simulink model "simulering_ROV_STA_controller"  (R2020a)
settings: Solver=ode45  StartTime=0.0  StopTime=t_sim  RelTol=1e-3
values from neighbouring files (symbols this model uses):
  alpha_los = atan2(y_los-y_start,x_los-x_start)    [run_simulation_SM_controller.m]    (also in run_simulation_STA_controller.m; run_simulation_dp_model.m)
  alpha_m_psi = 1    [run_simulation_STA_controller.m]    (also in tuning_STA_controller.m = 1.5)
  alpha_m_u = 1    [run_simulation_STA_controller.m]    (also in tuning_STA_controller.m = 1.5)
  alpha_m_v = 1    [run_simulation_STA_controller.m]    (also in tuning_STA_controller.m = 1.5)
  alpha_m_w = 1    [run_simulation_STA_controller.m]    (also in tuning_STA_controller.m = 1.5)
  B_aug = [b11 b12 b13 b14 b15 b16 ... (first row only)    [constants.m]
  B_psinv_aug = B_aug'/(B_aug*B_aug')    [constants.m]
  d_11 = 250    [constants.m]    (also in constants_dp_model.m; constants_model_coriolis.m; constants_process_model.m)
  d_22 = 200    [constants.m]    (also in constants_dp_model.m; constants_model_coriolis.m; constants_process_model.m)
  d_33 = 175    [constants.m]    (also in constants_dp_model.m; constants_model_coriolis.m; constants_process_model.m)
  d_66 = 15    [constants.m]    (also in constants_process_model.m)
  d_n11 = 350    [constants.m]
  d_n22 = 350    [constants.m]
  d_n33 = 400    [constants.m]
  d_n66 = 75    [constants.m]
  Delta = 25    [plot_simulation_feedback.m]    (also in run_simulation.m; run_simulation_SM_controller.m; run_simulation_STA_controller.m; run_simulation_dp_model.m)
  epsilon_psi = 1    [run_simulation_STA_controller.m]    (also in tuning_STA_controller.m = 0.0001)
  epsilon_u = 1    [run_simulation_STA_controller.m]    (also in tuning_STA_controller.m = 0.0001)
  epsilon_v = 1    [run_simulation_STA_controller.m]    (also in tuning_STA_controller.m = 0.0001)
  epsilon_w = 1    [run_simulation_STA_controller.m]    (also in tuning_STA_controller.m = 0.0001)
  g_z = 9.81    [run_simulation_FL_controller.m]    (also in run_simulation_PID_controller.m = 0.91; run_simulation_SM_controller.m = 0.91; run_simulation_STA_controller.m = 0.91; run_simulation_dp_model.m = 0.91)
  gam_psi = 1    [run_simulation_STA_controller.m]    (also in tuning_STA_controller.m)
  gam_u = 1    [run_simulation_STA_controller.m]    (also in tuning_STA_controller.m)
  gam_v = 1    [run_simulation_STA_controller.m]    (also in tuning_STA_controller.m)
  gam_w = 1    [run_simulation_STA_controller.m]    (also in tuning_STA_controller.m)
  gamma_r = 0.1    [run_simulation_FL_controller.m]    (also in run_simulation_PID_controller.m; run_simulation_SM_controller.m; run_simulation_STA_controller.m; run_simulation_feedback_linearizing.m)
  gamma_u = 0.1    [run_simulation_FL_controller.m]    (also in run_simulation_PID_controller.m; run_simulation_SM_controller.m; run_simulation_STA_controller.m; run_simulation_feedback_linearizing.m)
  gamma_v = 0.1    [run_simulation_FL_controller.m]    (also in run_simulation_PID_controller.m; run_simulation_SM_controller.m; run_simulation_STA_controller.m; run_simulation_feedback_linearizing.m)
  lambda = d_44    [run_simulation_FL_controller.m]    (also in run_simulation_PID_controller.m = 1; run_simulation_SM_controller.m = 1; run_simulation_STA_controller.m = 1; run_simulation_feedback_linearizing.m = 1)
  lambda_psi = 1    [run_simulation_SM_controller.m]    (also in run_simulation_STA_controller.m; tuning_SM_controller.m; tuning_STA_controller.m = 0.5)
  lambda_u = 0.5    [run_simulation_SM_controller.m]    (also in run_simulation_STA_controller.m = 1; tuning_SM_controller.m; tuning_STA_controller.m = 10)
  lambda_v = 0.5    [run_simulation_SM_controller.m]    (also in run_simulation_STA_controller.m = 1; tuning_SM_controller.m; tuning_STA_controller.m = 10)
  lambda_w = 1    [run_simulation_STA_controller.m]    (also in tuning_STA_controller.m = 0.5)
  m_11 = m_RB11+m_A11    (= 144)    [constants.m]    (also in constants_dp_model.m; constants_model_coriolis.m; constants_process_model.m)
  m_22 = m_RB22+m_A22    (= 162)    [constants.m]    (also in constants_dp_model.m; constants_model_coriolis.m; constants_process_model.m)
  m_66 = m_RB66+m_A66    (= 18.2)    [constants.m]    (also in constants_process_model.m)
  m_A11 = 54    [constants.m]    (also in constants_dp_model.m; constants_model_coriolis.m; constants_process_model.m)
  m_A22 = 72    [constants.m]    (also in constants_dp_model.m; constants_model_coriolis.m; constants_process_model.m)
  m_A33 = 360    [constants.m]    (also in constants_dp_model.m; constants_model_coriolis.m; constants_process_model.m)
  m_A66 = 5.2    [constants.m]    (also in constants_process_model.m)
  m_RB11 = 90    [constants.m]    (also in constants_dp_model.m; constants_model_coriolis.m; constants_process_model.m)
  m_RB22 = 90    [constants.m]    (also in constants_dp_model.m; constants_model_coriolis.m; constants_process_model.m)
  m_RB33 = 90    [constants.m]    (also in constants_dp_model.m; constants_model_coriolis.m; constants_process_model.m)
  m_RB66 = 13    [constants.m]    (also in constants_process_model.m)
  omega_psi = 1    [run_simulation_STA_controller.m]    (also in tuning_STA_controller.m = 0.001)
  omega_ref = 1.5    [run_simulation.m]    (also in run_simulation_FL_controller.m = 0.4; run_simulation_PID_controller.m = 0.4; run_simulation_SM_controller.m; run_simulation_STA_controller.m = 0.4)
  omega_u = 1    [run_simulation_STA_controller.m]    (also in tuning_STA_controller.m = 0.01)
  omega_v = 1    [run_simulation_STA_controller.m]    (also in tuning_STA_controller.m = 0.01)
  omega_w = 1    [run_simulation_STA_controller.m]    (also in tuning_STA_controller.m = 0.01)
  psi0 = deg2rad(psi0)    [constants.m]    (also in constants_dp_model.m; constants_model_coriolis.m; constants_process_model.m)
  r0 = 0    [constants.m]    (also in constants_dp_model.m; constants_model_coriolis.m; constants_process_model.m)
  T_ref = 0.2    [run_simulation.m]    (also in run_simulation_FL_controller.m; run_simulation_PID_controller.m; run_simulation_SM_controller.m; run_simulation_STA_controller.m)
  tau_r_max = sqrt(torque_co'*torque_co)    [constants.m]    (also in constants_dp_model.m; constants_model_coriolis.m; constants_process_model.m; run_simulation_feedback_linearizing.m = sqrt(torque_co'*torque_co)/(m_A33+m_RB33))
  tau_u_max = (F_max*cos(alpha1)+F_max*cos(alpha2)+F_max*cos(alpha3)+F_max*cos(alpha4))    [constants.m]    (also in constants_dp_model.m; constants_model_coriolis.m; constants_process_model.m; run_simulation_feedback_linearizing.m = (F_max*cos(alpha1)+F_max*cos(alpha2)+F_max*cos(alpha3)+F_max)
  tau_v_max = (F_max*sin(alpha1)-F_max*sin(alpha2)+F_max*sin(alpha3)-F_max*sin(alpha4))    [constants.m]    (also in constants_dp_model.m; constants_model_coriolis.m; constants_process_model.m; run_simulation_feedback_linearizing.m = (F_max*sin(alpha1)-F_max*sin(alpha2)+F_max*sin(alpha3)-F_max)
  tau_w_max = 2*F_max    (= 240)    [constants.m]    (also in constants_dp_model.m; constants_model_coriolis.m; constants_process_model.m)
  u0 = 0    [constants.m]    (also in constants_dp_model.m; constants_model_coriolis.m; constants_process_model.m)
  u_r = 0.14    [run_simulation.m]    (also in run_simulation_FL_controller.m = 0.2; run_simulation_PID_controller.m = 0.2; run_simulation_SM_controller.m; run_simulation_STA_controller.m = 0.2)
  v0 = 0    [constants.m]    (also in constants_dp_model.m; constants_model_coriolis.m; constants_process_model.m)
  v_r = 0.14    [run_simulation.m]    (also in run_simulation_FL_controller.m = 0; run_simulation_PID_controller.m = 0; run_simulation_SM_controller.m; run_simulation_STA_controller.m = 0)
  V_x_mat = load('Vx_disturbance.mat').u    [run_simulation_SM_controller.m]    (also in run_simulation_STA_controller.m; run_simulation_dp_model.m)
  V_y_mat = load('Vy_disturbance.mat').v    [run_simulation_SM_controller.m]    (also in run_simulation_STA_controller.m; run_simulation_dp_model.m)
  w0 = 0    [constants.m]    (also in constants_dp_model.m; constants_model_coriolis.m; constants_process_model.m)
  x0 = -2*50    (= -100)    [constants.m]    (also in constants_dp_model.m = 0; constants_model_coriolis.m = 0; constants_process_model.m = 0)
  x_start = -2*50    (= -100)    [plot_simulation_feedback.m]    (also in run_simulation_SM_controller.m; run_simulation_STA_controller.m; run_simulation_dp_model.m)
  y0 = 0    [constants.m]    (also in constants_dp_model.m; constants_model_coriolis.m; constants_process_model.m)
  y_start = 1*80    (= 80)    [plot_simulation_feedback.m]    (also in run_simulation_SM_controller.m; run_simulation_STA_controller.m = 50; run_simulation_dp_model.m)
  z0 = 0    [constants.m]    (also in constants_dp_model.m; constants_model_coriolis.m; constants_process_model.m)
  z_r = 10    [run_simulation.m]    (also in run_simulation_FL_controller.m = 1; run_simulation_PID_controller.m = 1; run_simulation_SM_controller.m; run_simulation_STA_controller.m = 1)
  zeta_ref = 1    [run_simulation.m]    (also in run_simulation_FL_controller.m; run_simulation_PID_controller.m; run_simulation_SM_controller.m; run_simulation_STA_controller.m)
settings Model: Creator=kenng  LastModifiedBy=kenng

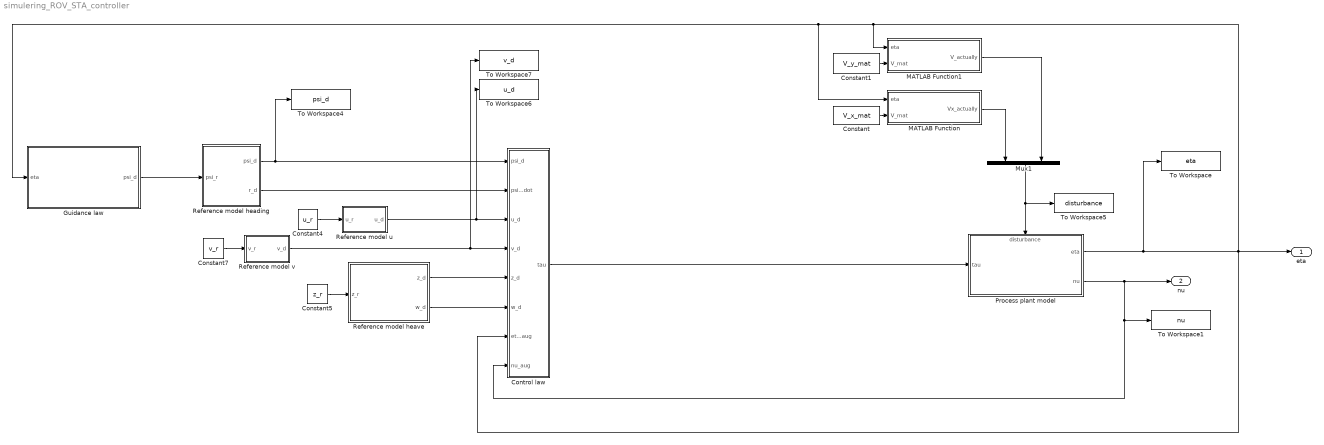
== system simulering_ROV_STA_controller ==
  Constant : Constant  Value=V_x_mat
  Constant1 : Constant  Value=V_y_mat
  Constant4 : Constant  Value=u_r
  Constant5 : Constant  Value=z_r
  Constant7 : Constant  Value=v_r
  Control law : Subsystem
  Guidance law : Subsystem
  MATLAB Function : MATLAB Function  TreatAsAtomicUnit=on
  MATLAB Function1 : MATLAB Function  TreatAsAtomicUnit=on
  Mux1 : Mux  Inputs=2
  Process plant model : Subsystem
      settings: PortSchema="{\"entries\":[{\"content\":{\"sides\":[{\"content\":{\"connectorIds\":[\"In1\"]},\"type\":\"ConnectorPlacement.EquallySpacedRectSide\",\"uuid\":\"e717a587-3200-458e-ba24-dd41565550b9\"},{\"content\":{\"connectorIds\":[\"Out1\",\"Out2\"],\"side\":\"RIGHT\"},\"type\":\"ConnectorPlacement.EquallySpacedRectSide\",\"uuid\":\"302c9cc9-c34e-45c2-bf93-40982187bd66\"},{\"content\":{\"connectorIds\":[\"In2\"],\"side\":\"TOP\"},\"type\":\"ConnectorPlacement.EquallySpacedRectSide\",\"uuid\":\"4b1c13ad-6fa1-447d-8a08-ad292496a8ea\"}]},\"type\":\"ConnectorPlacement.EquallySpacedConnector\",\"uuid\":\"78ff5622-69b9-4402-ac71-5e2cc2861626\"}],\"packageUris\":[\"http://schema.mathworks.com/mf0/Connector/19700101\"],\"version\":\"1.0\"}"
  Reference model heading : Subsystem
  Reference model heave : Subsystem
  Reference model u : Subsystem
  Reference model v : Subsystem
  To Workspace : ToWorkspace  VariableName=eta  SaveFormat=Structure With Time  SampleTime=-1
  To Workspace1 : ToWorkspace  VariableName=nu  SaveFormat=Structure With Time  SampleTime=-1
  To Workspace4 : ToWorkspace  VariableName=psi_d  SaveFormat=Structure With Time  SampleTime=-1
  To Workspace5 : ToWorkspace  VariableName=disturbance  SaveFormat=Structure With Time  SampleTime=-1
  To Workspace6 : ToWorkspace  VariableName=u_d  SaveFormat=Structure With Time  SampleTime=-1
  To Workspace7 : ToWorkspace  VariableName=v_d  SaveFormat=Structure With Time  SampleTime=-1
  eta : Outport
  nu : Outport  Port=2
  wires:
  Process plant model/2(nu) -> nu/1, To Workspace1/1, Control law/8(nu_aug)
  Mux1/1 -> Process plant model/2(disturbance), To Workspace5/1
  MATLAB Function/1(Vx_actually) -> Mux1/1
  MATLAB Function1/1(V_actually) -> Mux1/2
  Reference model heave/1(z_d) -> Control law/5(z_d)
  Reference model u/1(u_d) -> To Workspace6/1, Control law/3(u_d)
  Constant7/1 -> Reference model v/1(v_r)
  Guidance law/1(psi_d) -> Reference model heading/1(psi_r)
  Reference model heave/2(w_d) -> Control law/6(w_d)
  Reference model heading/1(psi_d) -> Control law/1(psi_d), To Workspace4/1
  Constant4/1 -> Reference model u/1(u_r)
  Reference model v/1(v_d) -> To Workspace7/1, Control law/4(v_d)
  Reference model heading/2(r_d) -> Control law/2(psi_d_dot)
  Constant5/1 -> Reference model heave/1(z_r)
  Control law/1(tau) -> Process plant model/1(tau)
  Constant1/1 -> MATLAB Function1/2(V_mat)
  Process plant model/1(eta) -> To Workspace/1, MATLAB Function1/1(eta), Guidance law/1(eta), MATLAB Function/1(eta), Control law/7(eta_aug), eta/1
  Constant/1 -> MATLAB Function/2(V_mat)

== system simulering_ROV_STA_controller/Control law ==
  psi_d : Inport
  psi_d_dot : Inport  Port=2
  u_d : Inport  Port=3
  v_d : Inport  Port=4
  z_d : Inport  Port=5
  w_d : Inport  Port=6
  eta_aug : Inport  Port=7
  nu_aug : Inport  Port=8
  Adaptive law r : Subsystem
  Adaptive law u : Subsystem
  Adaptive law v : Subsystem
  Heave controller : Subsystem
  Mux : Mux
  Surge controller : Subsystem
  Sway controller : Subsystem
  To Workspace : ToWorkspace  VariableName=V_yv_hat  SaveFormat=Structure With Time  SampleTime=-1
  To Workspace1 : ToWorkspace  VariableName=V_yu_hat  SaveFormat=Structure With Time  SampleTime=-1
  To Workspace2 : ToWorkspace  VariableName=V_xv_hat  SaveFormat=Structure With Time  SampleTime=-1
  To Workspace3 : ToWorkspace  VariableName=V_xu_hat  SaveFormat=Structure With Time  SampleTime=-1
  To Workspace4 : ToWorkspace  VariableName=V_xr_hat  SaveFormat=Structure With Time  SampleTime=-1
  To Workspace5 : ToWorkspace  VariableName=V_yr_hat  SaveFormat=Structure With Time  SampleTime=-1
  To Workspace6 : ToWorkspace  VariableName=V_xr_hat_sq  SaveFormat=Structure With Time  SampleTime=-1
  To Workspace7 : ToWorkspace  VariableName=V_yr_hat_sq  SaveFormat=Structure With Time  SampleTime=-1
  To Workspace8 : ToWorkspace  VariableName=V_xyr_hat  SaveFormat=Structure With Time  SampleTime=-1
  Yaw controller : Subsystem
  tau : Outport
  wires:
  Heave controller/1(tau_w) -> Mux/3
  Mux/1 -> tau/1
  u_d/1 -> Surge controller/1(u_d), Adaptive law u/3(u_d)
  v_d/1 -> Adaptive law v/3(v_d), Sway controller/1(v_d)
  z_d/1 -> Heave controller/1(z_d)
  Adaptive law u/2(V_y_u_hat) -> To Workspace1/1
  Adaptive law u/1(V_x_u_hat) -> To Workspace3/1
  Adaptive law v/1(V_yv_hat) -> To Workspace/1
  Adaptive law v/2(V_xv_hat) -> To Workspace2/1
  Adaptive law r/1(V_xr_hat) -> To Workspace4/1
  Adaptive law r/2(V_yr_hat) -> To Workspace5/1
  Adaptive law r/3(V_xr_hat_sq) -> To Workspace6/1
  Adaptive law r/4(V_yr_hat_sq) -> To Workspace7/1
  Adaptive law r/5(V_xyr_hat) -> To Workspace8/1
  [psi_d] -> Adaptive law r/3(psi_d)
  psi_d_dot/1 -> Yaw controller/4(psi_d_dot), Adaptive law r/4(psi_d_dot)
  eta_aug/1 -> Adaptive law u/1(eta), Adaptive law v/1(eta), Surge controller/3(eta), Sway controller/3(eta), Heave controller/4(eta), Adaptive law r/1(eta), Yaw controller/1(eta)
  nu_aug/1 -> Adaptive law r/2(nu), Yaw controller/2(nu), Heave controller/3(nu), Sway controller/2(nu), Adaptive law u/2(nu), Adaptive law v/2(nu), Surge controller/2(nu)
  psi_d/1 -> Yaw controller/3(psi_d), [psi_d]
  Yaw controller/1(tau_r) -> Mux/4
  Surge controller/1(tau_u) -> Mux/1
  Sway controller/1(tau_v) -> Mux/2
  w_d/1 -> Heave controller/2(w_d)

== system simulering_ROV_STA_controller/Guidance law ==
  eta : Inport
  Constant : Constant  Value=Delta
  Constant1 : Constant  Value=alpha_los
  Constant2 : Constant  Value=y_start
  Constant3 : Constant  Value=x_start
  Cos : Trigonometry  Operator=cos
  Demux : Demux
  Product : Product
  Product1 : Product
  Sin : Trigonometry
  Sum : Sum  Inputs=|-+
  Sum1 : Sum  Inputs=|+-
  Sum2 : Sum  Inputs=|-+
  Sum3 : Sum  Inputs=-+|
  Tan : Trigonometry  Operator=atan2
  Terminator : Terminator
  Terminator1 : Terminator
  psi_d : Outport
  wires:
  eta/1 -> Demux/1
  Demux/3 -> Terminator/1
  Demux/4 -> Terminator1/1
  Constant/1 -> Tan/2
  Sum/1 -> psi_d/1
  Constant1/1 -> Sum/2, Sin/1, Cos/1
  Tan/1 -> Sum/1
  Constant2/1 -> Sum1/2
  Demux/2 -> Sum1/1
  Cos/1 -> Product/2
  Sum1/1 -> Product/1
  Sin/1 -> Product1/2
  Demux/1 -> Sum2/2
  Constant3/1 -> Sum2/1
  Sum2/1 -> Product1/1
  Product/1 -> Sum3/2
  Product1/1 -> Sum3/1
  Sum3/1 -> Tan/1

== system simulering_ROV_STA_controller/Process plant model ==
  note: tau: 4x1 vector = [surge sway heave yaw]^T
  note: Disturbance: 3x1 vector = [Vx Vy gz]^t
  tau : Inport
  disturbance : Inport  Port=2
  Demux : Demux
  Kinematics : Subsystem
  Kinetics : Subsystem
  Terminator : Terminator
  Terminator1 : Terminator
  Terminator2 : Terminator
  Thruster saturation : Subsystem
  To Workspace2 : ToWorkspace  VariableName=tau_unsat  SaveFormat=Structure With Time  SampleTime=-1
  To Workspace3 : ToWorkspace  VariableName=tau_sat  SaveFormat=Structure With Time  SampleTime=-1
  eta : Outport
  nu : Outport  Port=2
  wires:
  Kinetics/1(nu) -> nu/1, Kinematics/1(nu)
  Demux/4 -> Kinetics/3(psi)
  Demux/2 -> Terminator1/1
  Kinematics/1(eta) -> eta/1, Demux/1
  Demux/1 -> Terminator/1
  Demux/3 -> Terminator2/1
  disturbance/1 -> Kinetics/1(disturbance)
  Thruster saturation/1(tau_sat) -> Kinetics/2(tau), To Workspace3/1
  tau/1 -> Thruster saturation/1(tau_unsat), To Workspace2/1

== system simulering_ROV_STA_controller/Reference model heading ==
  note: psi_r
  note: psi_d
  note: r_d
  note: a_d
  psi_r : Inport
  Gain : Gain  Gain=(2*zeta_ref+1)*omega_ref
  Gain1 : Gain  Gain=(2*zeta_ref+1)*omega_ref^2
  Gain2 : Gain  Gain=omega_ref^3
  Integrator : Integrator
  Integrator1 : Integrator
  Integrator2 : Integrator
  Saturation : Saturate  UpperLimit=tau_r_max/(m_RB11*0.2^2)  LowerLimit=-tau_r_max/(m_RB11*0.2^2)
  Sum : Sum  Inputs=|+-
  Sum1 : Sum  Inputs=-+|
  Sum2 : Sum  Inputs=-+|
  psi_d : Outport
  r_d : Outport  Port=2
  wires:
  Sum1/1 -> Integrator1/1
  Sum2/1 -> Gain2/1
  Integrator2/1 -> psi_d/1, Sum2/1
  Sum/1 -> Sum1/2
  Saturation/1 -> Gain/1, Integrator/1
  Integrator/1 -> r_d/1, Gain1/1, Integrator2/1
  Gain2/1 -> Sum/1
  Gain/1 -> Sum/2
  Gain1/1 -> Sum1/1
  Integrator1/1 -> Saturation/1
  psi_r/1 -> Sum2/2

== system simulering_ROV_STA_controller/Reference model heave ==
  note: z_r
  note: z_d
  note: w_d
  note: a_ud
  z_r : Inport
  Gain : Gain  Gain=(2*zeta_ref+1)*omega_ref
  Gain1 : Gain  Gain=(2*zeta_ref+1)*omega_ref^2
  Gain2 : Gain  Gain=omega_ref^3
  Integrator : Integrator
  Integrator1 : Integrator
  Integrator2 : Integrator
  Saturation : Saturate  UpperLimit=tau_w_max/m_RB11  LowerLimit=-tau_w_max/m_RB11
  Sum : Sum  Inputs=|+-
  Sum1 : Sum  Inputs=-+|
  Sum2 : Sum  Inputs=-+|
  z_d : Outport
  w_d : Outport  Port=2
  wires:
  Sum1/1 -> Integrator1/1
  Sum2/1 -> Gain2/1
  Integrator2/1 -> z_d/1, Sum2/1
  Sum/1 -> Sum1/2
  Saturation/1 -> Integrator/1, Gain/1
  Gain2/1 -> Sum/1
  Gain/1 -> Sum/2
  Gain1/1 -> Sum1/1
  Integrator1/1 -> Saturation/1
  z_r/1 -> Sum2/2
  Integrator/1 -> w_d/1, Gain1/1, Integrator2/1

== system simulering_ROV_STA_controller/Reference model u ==
  note: u_r
  u_r : Inport
  Gain : Gain  Gain=1/T_ref
  Integrator : Integrator
  Saturation : Saturate  UpperLimit=tau_u_max/m_RB11  LowerLimit=-tau_u_max/m_RB11
  Sum : Sum  Inputs=|+-
  u_d : Outport
  wires:
  u_r/1 -> Sum/1
  Sum/1 -> Gain/1
  Integrator/1 -> u_d/1, Sum/2
  Gain/1 -> Saturation/1
  Saturation/1 -> Integrator/1

== system simulering_ROV_STA_controller/Reference model v ==
  note: v_r
  v_r : Inport
  Gain : Gain  Gain=1/T_ref
  Integrator : Integrator
  Saturation1 : Saturate  UpperLimit=tau_v_max/m_RB11  LowerLimit=-tau_v_max/m_RB11
  Sum : Sum  Inputs=|+-
  v_d : Outport
  wires:
  v_r/1 -> Sum/1
  Sum/1 -> Gain/1
  Gain/1 -> Saturation1/1
  Integrator/1 -> v_d/1, Sum/2
  Saturation1/1 -> Integrator/1

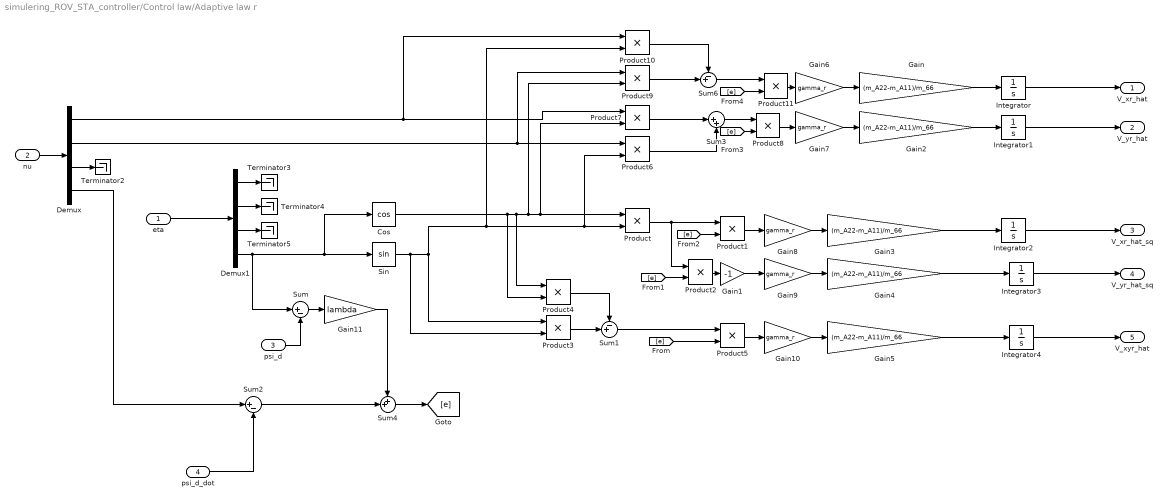
== system simulering_ROV_STA_controller/Control law/Adaptive law r ==
  eta : Inport
  nu : Inport  Port=2
  psi_d : Inport  Port=3
  psi_d_dot : Inport  Port=4
  Cos : Trigonometry  Operator=cos
  Demux : Demux
  Demux1 : Demux
  Gain{,2..5} (5 alike) : Gain  Gain=(m_A22-m_A11)/m_66
  Gain1 : Gain  Gain=-1
  Gain{6..10} (5 alike) : Gain  Gain=gamma_r
  Gain11 : Gain  Gain=lambda
  Integrator{,1..4} (5 alike) : Integrator
  Product{,1..11} (12 alike) : Product
  Sin : Trigonometry
  Sum : Sum  Inputs=|+-
  Sum1 : Sum  Inputs=-+|
  Sum2 : Sum  Inputs=|+-
  Sum3 : Sum  Inputs=|++
  Sum4 : Sum  Inputs=++|
  Sum6 : Sum  Inputs=-+|
  Terminator{2..5} (4 alike) : Terminator
  V_xr_hat : Outport
  V_yr_hat : Outport  Port=2
  V_xr_hat_sq : Outport  Port=3
  V_yr_hat_sq : Outport  Port=4
  V_xyr_hat : Outport  Port=5
  wires:
  [e] -> Product11/2
  [e] -> Product8/2
  nu/1 -> Demux/1
  Demux/1 -> Product10/1, Product7/1
  Demux/2 -> Product9/1, Product6/1
  Demux/3 -> Terminator2/1
  Demux1/2 -> Terminator4/1
  eta/1 -> Demux1/1
  Demux1/1 -> Terminator3/1
  Demux1/3 -> Terminator5/1
  Demux1/4 -> Cos/1, Sin/1, Sum/1
  Demux/4 -> Sum2/1
  Sin/1 -> Product3/2, Product3/1, Product10/2, Product6/2, Product/2
  Cos/1 -> Product4/2, Product4/1, Product9/2, Product7/2, Product/1
  [e] -> Product1/2
  Product1/1 -> Gain8/1
  Product2/1 -> Gain1/1
  [e] -> Product2/2
  Product/1 -> Product2/1, Product1/1
  Product3/1 -> Sum1/2
  Product4/1 -> Sum1/1
  Sum1/1 -> Product5/1
  [e] -> Product5/2
  Product7/1 -> Sum3/1
  Product6/1 -> Sum3/2
  Sum3/1 -> Product8/1
  Product9/1 -> Sum6/2
  Product10/1 -> Sum6/1
  Sum6/1 -> Product11/1
  Gain1/1 -> Gain9/1
  Product11/1 -> Gain6/1
  Product8/1 -> Gain7/1
  Product5/1 -> Gain10/1
  Gain/1 -> Integrator/1
  Gain2/1 -> Integrator1/1
  Gain3/1 -> Integrator2/1
  Gain4/1 -> Integrator3/1
  Gain5/1 -> Integrator4/1
  Integrator4/1 -> V_xyr_hat/1
  Integrator3/1 -> V_yr_hat_sq/1
  Integrator2/1 -> V_xr_hat_sq/1
  Integrator1/1 -> V_yr_hat/1
  Integrator/1 -> V_xr_hat/1
  Gain6/1 -> Gain/1
  Gain7/1 -> Gain2/1
  Gain8/1 -> Gain3/1
  Gain9/1 -> Gain4/1
  Gain10/1 -> Gain5/1
  psi_d_dot/1 -> Sum2/2
  psi_d/1 -> Sum/2
  Sum/1 -> Gain11/1
  Sum2/1 -> Sum4/2
  Gain11/1 -> Sum4/1
  Sum4/1 -> [e]

== system simulering_ROV_STA_controller/Control law/Adaptive law u ==
  eta : Inport
  nu : Inport  Port=2
  u_d : Inport  Port=3
  Cos : Trigonometry  Operator=cos
  Demux : Demux
  Demux1 : Demux
  Gain : Gain  Gain=d_11/m_11
  Gain1 : Gain  Gain=d_11/m_11
  Gain2 : Gain  Gain=(m_A11-m_A22)/m_11
  Gain3 : Gain  Gain=(m_A11-m_A22)/m_11
  Gain4 : Gain  Gain=gamma_u
  Integrator : Integrator
  Integrator1 : Integrator
  Product{,1..3} (4 alike) : Product
  Sin : Trigonometry
  Sum : Sum  Inputs=-+|
  Sum1 : Sum  Inputs=-+|
  Sum2 : Sum  Inputs=|++
  Terminator{1..5} (5 alike) : Terminator
  V_x_u_hat : Outport
  V_y_u_hat : Outport  Port=2
  wires:
  Sin/1 -> Product2/2, Gain1/1
  Product/1 -> Integrator/1
  Product1/1 -> Integrator1/1
  Gain4/1 -> Product1/2, Product/1
  Integrator/1 -> V_x_u_hat/1
  Gain/1 -> Sum1/2
  Sum1/1 -> Product/2
  Gain2/1 -> Sum1/1
  nu/1 -> Demux/1
  Product2/1 -> Gain2/1
  Sum2/1 -> Product1/1
  Gain1/1 -> Sum2/1
  Product3/1 -> Gain3/1
  Cos/1 -> Product3/1, Gain/1
  Gain3/1 -> Sum2/2
  Demux/4 -> Product2/1, Product3/2
  Demux/1 -> Sum/2
  Demux/2 -> Terminator1/1
  Demux/3 -> Terminator2/1
  Demux1/2 -> Terminator4/1
  eta/1 -> Demux1/1
  Demux1/1 -> Terminator3/1
  Demux1/3 -> Terminator5/1
  Demux1/4 -> Cos/1, Sin/1
  u_d/1 -> Sum/1
  Sum/1 -> Gain4/1
  Integrator1/1 -> V_y_u_hat/1

== system simulering_ROV_STA_controller/Control law/Adaptive law v ==
  eta : Inport
  nu : Inport  Port=2
  v_d : Inport  Port=3
  Cos1 : Trigonometry  Operator=cos
  Demux : Demux
  Demux1 : Demux
  Gain : Gain  Gain=gamma_v
  Gain2 : Gain  Gain=d_22/m_22
  Gain3 : Gain  Gain=d_22/m_22
  Gain4 : Gain  Gain=(m_A11-m_A22)/m_22
  Gain5 : Gain  Gain=(m_A11-m_A22)/m_22
  Integrator : Integrator
  Integrator1 : Integrator
  Product{2..5} (4 alike) : Product
  Sin1 : Trigonometry
  Sum : Sum  Inputs=-+|
  Sum2 : Sum  Inputs=-+|
  Sum3 : Sum  Inputs=|--
  Terminator{,2..5} (5 alike) : Terminator
  V_yv_hat : Outport
  V_xv_hat : Outport  Port=2
  wires:
  Gain4/1 -> Sum2/1
  Product5/1 -> Gain5/1
  Gain2/1 -> Sum2/2
  Demux/3 -> Terminator2/1
  Product4/1 -> Gain4/1
  nu/1 -> Demux/1
  Gain5/1 -> Sum3/2
  Sum2/1 -> Product2/2
  Integrator1/1 -> V_yv_hat/1
  Gain/1 -> Product3/2, Product2/1
  Product2/1 -> Integrator1/1
  Sum3/1 -> Product3/1
  Demux/2 -> Sum/2
  Demux/1 -> Terminator/1
  Gain3/1 -> Sum3/1
  Demux/4 -> Product4/1, Product5/2
  Cos1/1 -> Product5/1, Gain2/1
  Sin1/1 -> Product4/2, Gain3/1
  Demux1/1 -> Terminator3/1
  Demux1/2 -> Terminator4/1
  eta/1 -> Demux1/1
  Demux1/3 -> Terminator5/1
  Demux1/4 -> Cos1/1, Sin1/1
  Product3/1 -> Integrator/1
  Integrator/1 -> V_xv_hat/1
  v_d/1 -> Sum/1
  Sum/1 -> Gain/1

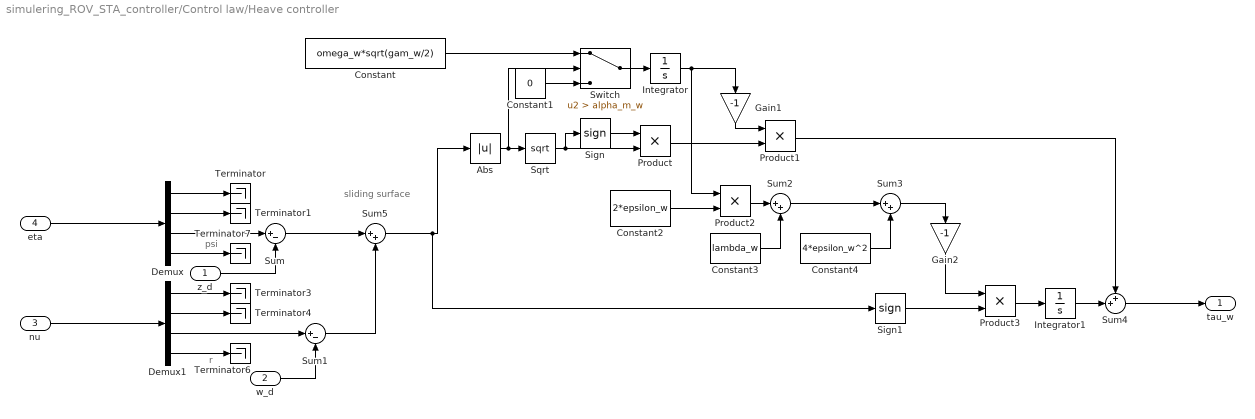
== system simulering_ROV_STA_controller/Control law/Heave controller ==
  note: r
  note: psi
  note: sliding surface
  z_d : Inport
  w_d : Inport  Port=2
  nu : Inport  Port=3
  eta : Inport  Port=4
  Abs : Abs
  Constant : Constant  Value=omega_w*sqrt(gam_w/2)
  Constant1 : Constant  Value=0
  Constant2 : Constant  Value=2*epsilon_w
  Constant3 : Constant  Value=lambda_w
  Constant4 : Constant  Value=4*epsilon_w^2
  Demux : Demux
  Demux1 : Demux
  Gain1 : Gain  Gain=-1
  Gain2 : Gain  Gain=-1
  Integrator : Integrator
  Integrator1 : Integrator
  Product{,1..3} (4 alike) : Product
  Sign : Signum
  Sign1 : Signum
  Sqrt : Sqrt  SaturateOnIntegerOverflow=on
  Sum : Sum  Inputs=|+-
  Sum1 : Sum  Inputs=|+-
  Sum2 : Sum  Inputs=|++
  Sum3 : Sum  Inputs=|++
  Sum4 : Sum  Inputs=++|
  Sum5 : Sum  Inputs=|++
  Switch : Switch  Criteria=u2 > Threshold  Threshold=alpha_m_w
  Terminator{,1,3..4,6..7} (6 alike) : Terminator
  tau_w : Outport
  wires:
  Demux1/2 -> Terminator4/1
  Demux/1 -> Terminator/1
  eta/1 -> Demux/1
  Demux/2 -> Terminator1/1
  Demux1/1 -> Terminator3/1
  Demux/3 -> Sum/1
  nu/1 -> Demux1/1
  Demux1/4 -> Terminator6/1
  Demux/4 -> Terminator7/1
  z_d/1 -> Sum/2
  Demux1/3 -> Sum1/1
  w_d/1 -> Sum1/2
  Integrator/1 -> Product2/1, Gain1/1
  Product2/1 -> Sum2/1
  Constant1/1 -> Switch/3
  Constant3/1 -> Sum2/2
  Product3/1 -> Integrator1/1
  Product1/1 -> Sum4/1
  Sign/1 -> Product/1
  Gain2/1 -> Product3/1
  Constant/1 -> Switch/1
  Gain1/1 -> Product1/1
  Constant4/1 -> Sum3/2
  Constant2/1 -> Product2/2
  Switch/1 -> Integrator/1
  Sum3/1 -> Gain2/1
  Sqrt/1 -> Sign/1, Product/2
  Sum2/1 -> Sum3/1
  Abs/1 -> Switch/2, Sqrt/1
  Integrator1/1 -> Sum4/2
  Sum4/1 -> tau_w/1
  Product/1 -> Product1/2
  Sign1/1 -> Product3/2
  Sum/1 -> Sum5/1
  Sum5/1 -> Sign1/1, Abs/1
  Sum1/1 -> Sum5/2

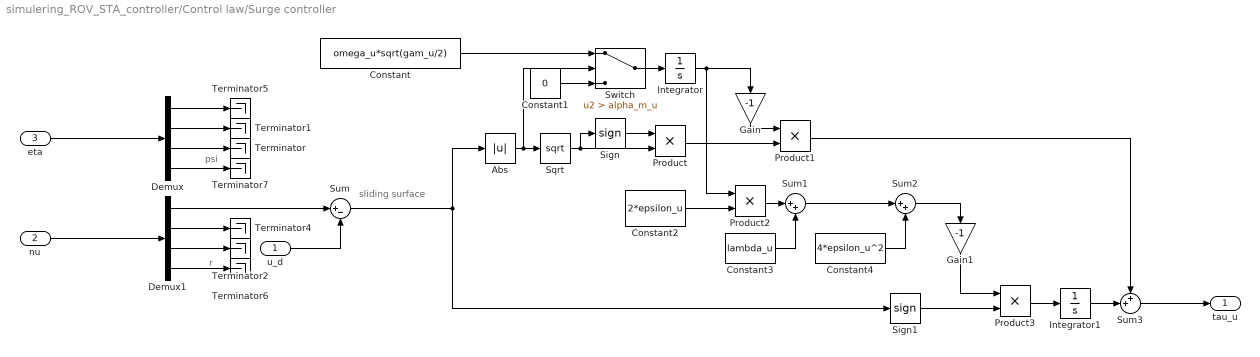
== system simulering_ROV_STA_controller/Control law/Surge controller ==
  note: sliding surface
  note: r
  note: psi
  u_d : Inport
  nu : Inport  Port=2
  eta : Inport  Port=3
  Abs : Abs
  Constant : Constant  Value=omega_u*sqrt(gam_u/2)
  Constant1 : Constant  Value=0
  Constant2 : Constant  Value=2*epsilon_u
  Constant3 : Constant  Value=lambda_u
  Constant4 : Constant  Value=4*epsilon_u^2
  Demux : Demux
  Demux1 : Demux
  Gain : Gain  Gain=-1
  Gain1 : Gain  Gain=-1
  Integrator : Integrator
  Integrator1 : Integrator
  Product{,1..3} (4 alike) : Product
  Sign : Signum
  Sign1 : Signum
  Sqrt : Sqrt  SaturateOnIntegerOverflow=on
  Sum : Sum  Inputs=|+-
  Sum1 : Sum  Inputs=|++
  Sum2 : Sum  Inputs=|++
  Sum3 : Sum  Inputs=++|
  Switch : Switch  Criteria=u2 > Threshold  Threshold=alpha_m_u
  Terminator{,1..2,4..7} (7 alike) : Terminator
  tau_u : Outport
  wires:
  Demux1/2 -> Terminator4/1
  eta/1 -> Demux/1
  Demux/2 -> Terminator1/1
  Demux1/1 -> Sum/1
  nu/1 -> Demux1/1
  Demux1/4 -> Terminator6/1
  Demux/4 -> Terminator7/1
  u_d/1 -> Sum/2
  Demux1/3 -> Terminator2/1
  Demux/3 -> Terminator/1
  Demux/1 -> Terminator5/1
  Sum/1 -> Sign1/1, Abs/1
  Abs/1 -> Switch/2, Sqrt/1
  Sqrt/1 -> Sign/1, Product/2
  Sign/1 -> Product/1
  Constant1/1 -> Switch/3
  Constant/1 -> Switch/1
  Product/1 -> Product1/2
  Switch/1 -> Integrator/1
  Integrator/1 -> Product2/1, Gain/1
  Gain/1 -> Product1/1
  Constant2/1 -> Product2/2
  Product2/1 -> Sum1/1
  Constant3/1 -> Sum1/2
  Sum1/1 -> Sum2/1
  Constant4/1 -> Sum2/2
  Sign1/1 -> Product3/2
  Sum2/1 -> Gain1/1
  Gain1/1 -> Product3/1
  Product3/1 -> Integrator1/1
  Integrator1/1 -> Sum3/2
  Product1/1 -> Sum3/1
  Sum3/1 -> tau_u/1

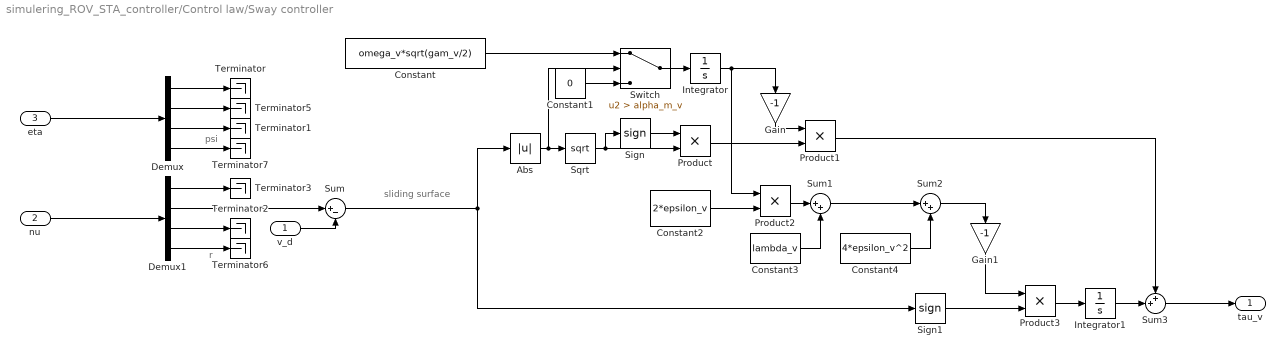
== system simulering_ROV_STA_controller/Control law/Sway controller ==
  note: r
  note: psi
  note: sliding surface
  v_d : Inport
  nu : Inport  Port=2
  eta : Inport  Port=3
  Abs : Abs
  Constant : Constant  Value=omega_v*sqrt(gam_v/2)
  Constant1 : Constant  Value=0
  Constant2 : Constant  Value=2*epsilon_v
  Constant3 : Constant  Value=lambda_v
  Constant4 : Constant  Value=4*epsilon_v^2
  Demux : Demux
  Demux1 : Demux
  Gain : Gain  Gain=-1
  Gain1 : Gain  Gain=-1
  Integrator : Integrator
  Integrator1 : Integrator
  Product{,1..3} (4 alike) : Product
  Sign : Signum
  Sign1 : Signum
  Sqrt : Sqrt  SaturateOnIntegerOverflow=on
  Sum : Sum  Inputs=|+-
  Sum1 : Sum  Inputs=|++
  Sum2 : Sum  Inputs=|++
  Sum3 : Sum  Inputs=++|
  Switch : Switch  Criteria=u2 > Threshold  Threshold=alpha_m_v
  Terminator{,1..3,5..7} (7 alike) : Terminator
  tau_v : Outport
  wires:
  Demux1/2 -> Sum/1
  Demux/1 -> Terminator/1
  eta/1 -> Demux/1
  Demux1/1 -> Terminator3/1
  nu/1 -> Demux1/1
  Demux1/4 -> Terminator6/1
  Demux/4 -> Terminator7/1
  v_d/1 -> Sum/2
  Demux1/3 -> Terminator2/1
  Demux/3 -> Terminator1/1
  Demux/2 -> Terminator5/1
  Integrator/1 -> Product2/1, Gain/1
  Product2/1 -> Sum1/1
  Constant1/1 -> Switch/3
  Constant3/1 -> Sum1/2
  Product3/1 -> Integrator1/1
  Product1/1 -> Sum3/1
  Sign/1 -> Product/1
  Gain1/1 -> Product3/1
  Constant/1 -> Switch/1
  Gain/1 -> Product1/1
  Constant4/1 -> Sum2/2
  Constant2/1 -> Product2/2
  Switch/1 -> Integrator/1
  Sum2/1 -> Gain1/1
  Sqrt/1 -> Sign/1, Product/2
  Sum1/1 -> Sum2/1
  Abs/1 -> Switch/2, Sqrt/1
  Integrator1/1 -> Sum3/2
  Sum3/1 -> tau_v/1
  Product/1 -> Product1/2
  Sign1/1 -> Product3/2
  Sum/1 -> Sign1/1, Abs/1

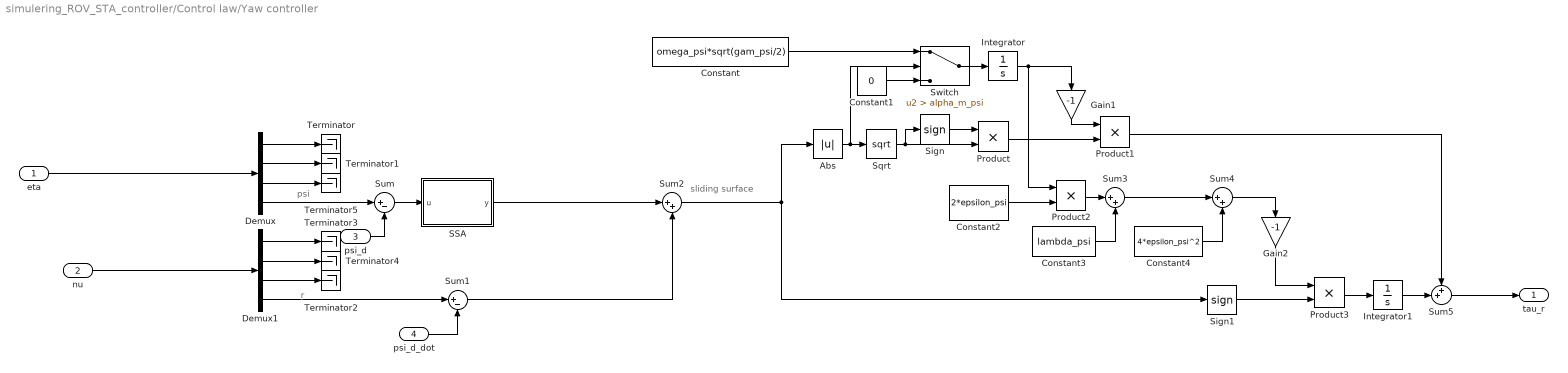
== system simulering_ROV_STA_controller/Control law/Yaw controller ==
  note: r
  note: psi
  note: sliding surface
  eta : Inport
  nu : Inport  Port=2
  psi_d : Inport  Port=3
  psi_d_dot : Inport  Port=4
  Abs : Abs
  Constant : Constant  Value=omega_psi*sqrt(gam_psi/2)
  Constant1 : Constant  Value=0
  Constant2 : Constant  Value=2*epsilon_psi
  Constant3 : Constant  Value=lambda_psi
  Constant4 : Constant  Value=4*epsilon_psi^2
  Demux : Demux
  Demux1 : Demux
  Gain1 : Gain  Gain=-1
  Gain2 : Gain  Gain=-1
  Integrator : Integrator
  Integrator1 : Integrator
  Product{,1..3} (4 alike) : Product
  SSA : MATLAB Function  TreatAsAtomicUnit=on
  Sign : Signum
  Sign1 : Signum
  Sqrt : Sqrt  SaturateOnIntegerOverflow=on
  Sum : Sum  Inputs=|+-
  Sum1 : Sum  Inputs=|+-
  Sum2 : Sum  Inputs=|++
  Sum3 : Sum  Inputs=|++
  Sum4 : Sum  Inputs=|++
  Sum5 : Sum  Inputs=++|
  Switch : Switch  Criteria=u2 > Threshold  Threshold=alpha_m_psi
  Terminator{,1..5} (6 alike) : Terminator
  tau_r : Outport
  wires:
  Demux/2 -> Terminator1/1
  Demux/1 -> Terminator/1
  Demux1/1 -> Terminator3/1
  Demux1/3 -> Terminator2/1
  Demux1/2 -> Terminator4/1
  eta/1 -> Demux/1
  nu/1 -> Demux1/1
  Demux/3 -> Terminator5/1
  psi_d/1 -> Sum/2
  Demux/4 -> Sum/1
  Demux1/4 -> Sum1/1
  psi_d_dot/1 -> Sum1/2
  Sum/1 -> SSA/1(u)
  SSA/1(y) -> Sum2/1
  Sum1/1 -> Sum2/2
  Integrator/1 -> Product2/1, Gain1/1
  Product2/1 -> Sum3/1
  Constant1/1 -> Switch/3
  Constant3/1 -> Sum3/2
  Product3/1 -> Integrator1/1
  Product1/1 -> Sum5/1
  Sign/1 -> Product/1
  Gain2/1 -> Product3/1
  Constant/1 -> Switch/1
  Gain1/1 -> Product1/1
  Constant4/1 -> Sum4/2
  Constant2/1 -> Product2/2
  Switch/1 -> Integrator/1
  Sum4/1 -> Gain2/1
  Sqrt/1 -> Sign/1, Product/2
  Sum3/1 -> Sum4/1
  Abs/1 -> Switch/2, Sqrt/1
  Integrator1/1 -> Sum5/2
  Sum5/1 -> tau_r/1
  Product/1 -> Product1/2
  Sign1/1 -> Product3/2
  Sum2/1 -> Sign1/1, Abs/1

== system simulering_ROV_STA_controller/Process plant model/Kinematics ==
  nu : Inport
  Cos : Trigonometry  Operator=cos
  Demux : Demux
  Integrator : Integrator  InitialCondition=psi0
  Integrator1 : Integrator  InitialCondition=z0
  Integrator2 : Integrator  InitialCondition=x0
  Integrator3 : Integrator  InitialCondition=y0
  Mux : Mux
  Product{,1..3} (4 alike) : Product
  Sin : Trigonometry
  Sum : Sum  Inputs=|++
  Sum1 : Sum  Inputs=|+-
  eta : Outport
  wires:
  Sin/1 -> [sinpsi]
  Demux/3 -> Integrator1/1
  Demux/1 -> Product1/1, Product/1
  Demux/2 -> Product3/1, Product2/1
  [sinpsi] -> Product3/2
  [psi] -> Sin/1, Cos/1
  [cospsi] -> Product2/2
  Cos/1 -> [cospsi]
  Product1/1 -> Sum/1
  Integrator/1 -> Mux/4, [psi]
  [sinpsi] -> Product1/2
  Product/1 -> Sum1/1
  Sum1/1 -> Integrator2/1
  Demux/4 -> Integrator/1
  Sum/1 -> Integrator3/1
  [cospsi] -> Product/2
  nu/1 -> Demux/1
  Product2/1 -> Sum/2
  Product3/1 -> Sum1/2
  Integrator3/1 -> Mux/2
  Integrator1/1 -> Mux/3
  Integrator2/1 -> Mux/1
  Mux/1 -> eta/1

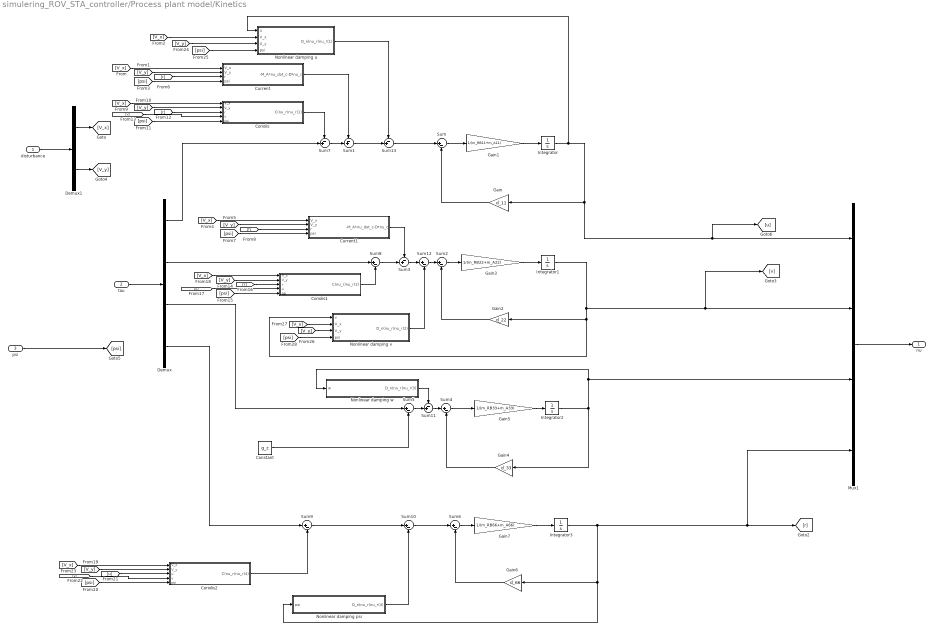
== system simulering_ROV_STA_controller/Process plant model/Kinetics ==
  disturbance : Inport
  tau : Inport  Port=2
  psi : Inport  Port=3
  Constant : Constant  Value=g_z
  Coriolis : Subsystem
  Coriolis1 : Subsystem
  Coriolis2 : Subsystem
  Current : Subsystem
  Current1 : Subsystem
  Demux : Demux
  Demux1 : Demux  Outputs=2
  Gain : Gain  Gain=d_11
  Gain1 : Gain  Gain=1/(m_RB11+m_A11)
  Gain2 : Gain  Gain=d_22
  Gain3 : Gain  Gain=1/(m_RB22+m_A22)
  Gain4 : Gain  Gain=d_33
  Gain5 : Gain  Gain=1/(m_RB33+m_A33)
  Gain6 : Gain  Gain=d_66
  Gain7 : Gain  Gain=1/(m_RB66+m_A66)
  Integrator : Integrator  InitialCondition=u0
  Integrator1 : Integrator  InitialCondition=v0
  Integrator2 : Integrator  InitialCondition=w0
  Integrator3 : Integrator  InitialCondition=r0
  Mux1 : Mux
  Nonlinear damping psi : Subsystem
  Nonlinear damping u : Subsystem
  Nonlinear damping v : Subsystem
  Nonlinear damping w : Subsystem
  Sum{,2,4..6,8..10,12} (9 alike) : Sum  Inputs=|+-
  Sum{1,3,7,11,13} (5 alike) : Sum  Inputs=-+|
  nu : Outport
  wires:
  Demux1/1 -> [V_x]
  Gain1/1 -> Integrator/1
  Sum/1 -> Gain1/1
  tau/1 -> Demux/1
  Integrator1/1 -> Gain2/1, Nonlinear damping v/1(v), [v], Mux1/2
  Gain3/1 -> Integrator1/1
  Mux1/1 -> nu/1
  Integrator/1 -> Nonlinear damping u/1(u), [u], Mux1/1, Gain/1
  Integrator2/1 -> Gain4/1, Nonlinear damping w/1(w), Mux1/3
  Gain5/1 -> Integrator2/1
  Sum4/1 -> Gain5/1
  Gain2/1 -> Sum2/2
  Sum2/1 -> Gain3/1
  Gain/1 -> Sum/2
  Gain4/1 -> Sum4/2
  Gain6/1 -> Sum6/2
  Demux1/2 -> [V_y]
  [r] -> Current/3(r)
  Integrator3/1 -> [r], Mux1/4, Nonlinear damping psi/1(psi), Gain6/1
  disturbance/1 -> Demux1/1
  Sum6/1 -> Gain7/1
  Gain7/1 -> Integrator3/1
  psi/1 -> [psi]
  Current/1(-M_A*nu_dot_c-D*nu_c) -> Sum1/1
  [V_y] -> Current/2(V_y)
  [V_x] -> Current/1(V_x)
  [psi] -> Current/4(psi)
  [r] -> Current1/3(r)
  [psi] -> Current1/4(psi)
  [V_x] -> Current1/1(V_x)
  [V_y] -> Current1/2(V_y)
  Current1/1(-M_A*nu_dot_c-D*nu_c) -> Sum3/1
  Constant/1 -> Sum5/2
  Demux/3 -> Sum5/1
  Coriolis/1(C(nu_r)nu_r(1)) -> Sum7/1
  Demux/1 -> Sum7/2
  Sum7/1 -> Sum1/2
  [V_x] -> Coriolis/1(V_x)
  [psi] -> Coriolis/5(psi)
  [r] -> Coriolis/3(r)
  [V_y] -> Coriolis/2(V_y)
  [v] -> Coriolis/4(v)
  [u] -> Coriolis1/4(u)
  Coriolis1/1(C(nu_r)nu_r(2)) -> Sum8/2
  [V_y] -> Coriolis1/2(V_y)
  [psi] -> Coriolis1/5(psi)
  [V_x] -> Coriolis1/1(V_x)
  [r] -> Coriolis1/3(r)
  Sum8/1 -> Sum3/2
  Demux/2 -> Sum8/1
  [v] -> Coriolis2/4(v)
  Coriolis2/1(C(nu_r)nu_r(4)) -> Sum9/2
  [V_y] -> Coriolis2/2(V_y)
  [psi] -> Coriolis2/5(psi)
  [V_x] -> Coriolis2/1(V_x)
  [u] -> Coriolis2/3(u)
  Demux/4 -> Sum9/1
  Sum10/1 -> Sum6/1
  Sum5/1 -> Sum11/2
  Sum11/1 -> Sum4/1
  Nonlinear damping w/1(D_n(nu_r)nu_r(3)) -> Sum11/1
  Sum12/1 -> Sum2/1
  Sum1/1 -> Sum13/2
  Sum13/1 -> Sum/1
  Nonlinear damping u/1(D_n(nu_r)nu_r(1)) -> Sum13/1
  [V_x] -> Nonlinear damping u/2(V_x)
  [V_y] -> Nonlinear damping u/3(V_y)
  [psi] -> Nonlinear damping u/4(psi)
  Sum3/1 -> Sum12/1
  Nonlinear damping v/1(D_n(nu_r)nu_r(2)) -> Sum12/2
  [V_x] -> Nonlinear damping v/2(V_x)
  [V_y] -> Nonlinear damping v/3(V_y)
  [psi] -> Nonlinear damping v/4(psi)
  Sum9/1 -> Sum10/1
  Nonlinear damping psi/1(D_n(nu_r)nu_r(4)) -> Sum10/2

== system simulering_ROV_STA_controller/Process plant model/Thruster saturation ==
  tau_unsat : Inport
  Constant : Constant  Value=B_psinv_aug
  Constant1 : Constant  Value=B_aug
  Demux : Demux  Outputs=6
  Matrix Multiply : Product  Multiplication=Matrix(*)
  Matrix Multiply1 : Product  Multiplication=Matrix(*)
  Mux : Mux  Inputs=6
  Saturation{,1..5} (6 alike) : Saturate  UpperLimit=120  LowerLimit=-120
  tau_sat : Outport
  wires:
  tau_unsat/1 -> Matrix Multiply/2
  Constant/1 -> Matrix Multiply/1
  Matrix Multiply/1 -> Demux/1
  Demux/2 -> Saturation1/1
  Demux/1 -> Saturation/1
  Demux/3 -> Saturation2/1
  Demux/4 -> Saturation3/1
  Demux/5 -> Saturation4/1
  Demux/6 -> Saturation5/1
  Saturation/1 -> Mux/1
  Saturation1/1 -> Mux/2
  Saturation2/1 -> Mux/3
  Saturation3/1 -> Mux/4
  Saturation4/1 -> Mux/5
  Saturation5/1 -> Mux/6
  Mux/1 -> Matrix Multiply1/2
  Constant1/1 -> Matrix Multiply1/1
  Matrix Multiply1/1 -> tau_sat/1

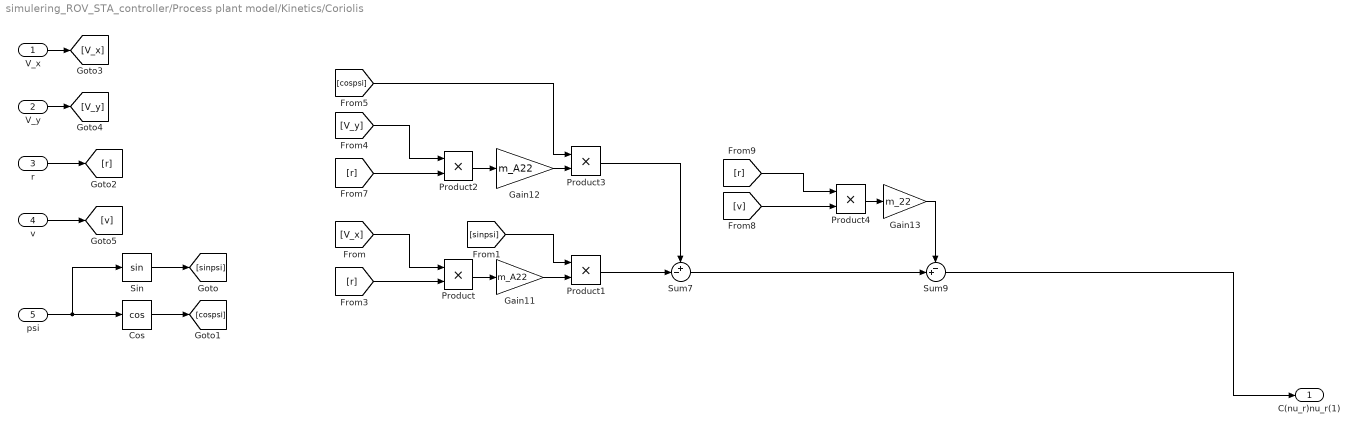
== system simulering_ROV_STA_controller/Process plant model/Kinetics/Coriolis ==
  V_x : Inport
  V_y : Inport  Port=2
  r : Inport  Port=3
  v : Inport  Port=4
  psi : Inport  Port=5
  Cos : Trigonometry  Operator=cos
  Gain11 : Gain  Gain=m_A22
  Gain12 : Gain  Gain=m_A22
  Gain13 : Gain  Gain=m_22
  Product{,1..4} (5 alike) : Product
  Sin : Trigonometry
  Sum7 : Sum  Inputs=+-|
  Sum9 : Sum  Inputs=-+|
  C(nu_r)nu_r(1) : Outport
  wires:
  Gain11/1 -> Product1/2
  Product2/1 -> Gain12/1
  [cospsi] -> Product3/1
  [r] -> Product2/2
  [v] -> Product4/2
  Product4/1 -> Gain13/1
  [V_x] -> Product/1
  Product3/1 -> Sum7/1
  Gain12/1 -> Product3/2
  Product/1 -> Gain11/1
  [V_y] -> Product2/1
  [r] -> Product/2
  Product1/1 -> Sum7/2
  [sinpsi] -> Product1/1
  Sum7/1 -> Sum9/2
  [r] -> Product4/1
  Sum9/1 -> C(nu_r)nu_r(1)/1
  psi/1 -> Sin/1, Cos/1
  Sin/1 -> [sinpsi]
  Cos/1 -> [cospsi]
  r/1 -> [r]
  V_x/1 -> [V_x]
  V_y/1 -> [V_y]
  v/1 -> [v]
  Gain13/1 -> Sum9/1

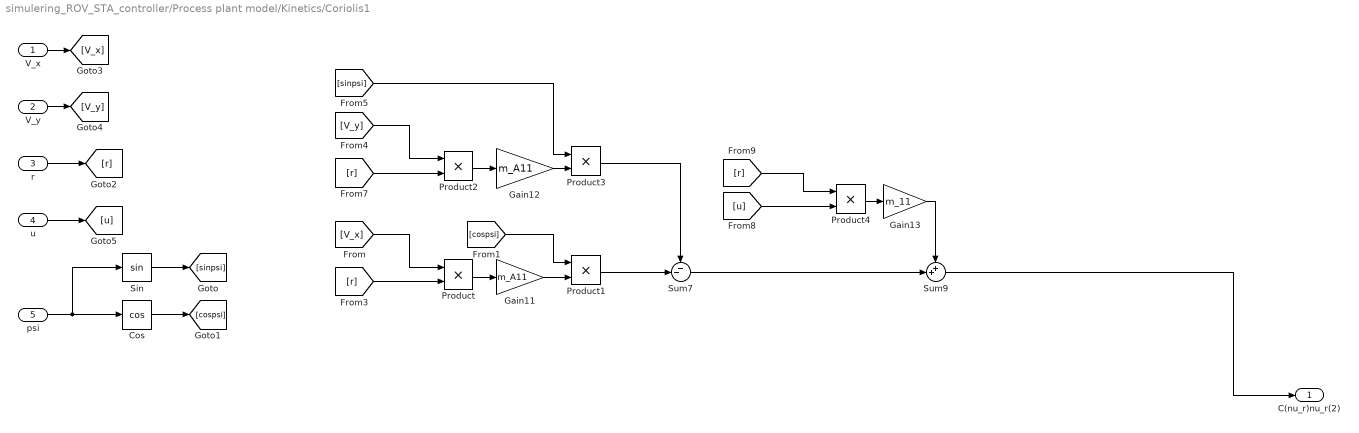
== system simulering_ROV_STA_controller/Process plant model/Kinetics/Coriolis1 ==
  V_x : Inport
  V_y : Inport  Port=2
  r : Inport  Port=3
  u : Inport  Port=4
  psi : Inport  Port=5
  Cos : Trigonometry  Operator=cos
  Gain11 : Gain  Gain=m_A11
  Gain12 : Gain  Gain=m_A11
  Gain13 : Gain  Gain=m_11
  Product{,1..4} (5 alike) : Product
  Sin : Trigonometry
  Sum7 : Sum  Inputs=--|
  Sum9 : Sum  Inputs=++|
  C(nu_r)nu_r(2) : Outport
  wires:
  Gain11/1 -> Product1/2
  Product2/1 -> Gain12/1
  [sinpsi] -> Product3/1
  [r] -> Product2/2
  [u] -> Product4/2
  Product4/1 -> Gain13/1
  [V_x] -> Product/1
  Product3/1 -> Sum7/1
  Gain12/1 -> Product3/2
  Product/1 -> Gain11/1
  [V_y] -> Product2/1
  [r] -> Product/2
  Product1/1 -> Sum7/2
  [cospsi] -> Product1/1
  Sum7/1 -> Sum9/2
  [r] -> Product4/1
  Sum9/1 -> C(nu_r)nu_r(2)/1
  psi/1 -> Sin/1, Cos/1
  Sin/1 -> [sinpsi]
  Cos/1 -> [cospsi]
  r/1 -> [r]
  V_x/1 -> [V_x]
  V_y/1 -> [V_y]
  u/1 -> [u]
  Gain13/1 -> Sum9/1

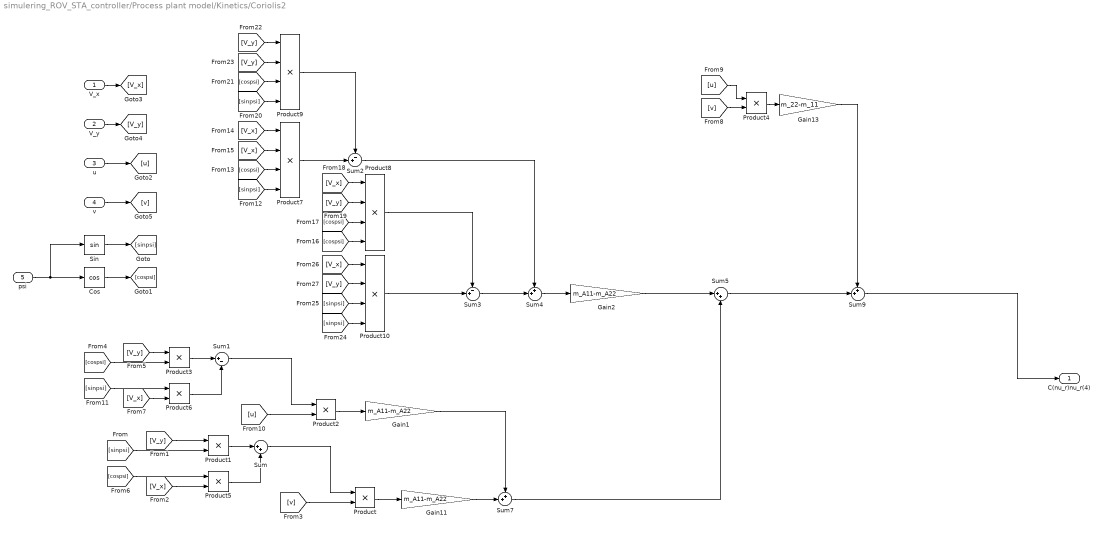
== system simulering_ROV_STA_controller/Process plant model/Kinetics/Coriolis2 ==
  V_x : Inport
  V_y : Inport  Port=2
  u : Inport  Port=3
  v : Inport  Port=4
  psi : Inport  Port=5
  Cos : Trigonometry  Operator=cos
  Gain1 : Gain  Gain=m_A11-m_A22
  Gain11 : Gain  Gain=m_A11-m_A22
  Gain13 : Gain  Gain=m_22-m_11
  Gain2 : Gain  Gain=m_A11-m_A22
  Product{,1..6} (7 alike) : Product
  Product{7..10} (4 alike) : Product  Inputs=4
  Sin : Trigonometry
  Sum : Sum  Inputs=|++
  Sum1 : Sum  Inputs=|+-
  Sum2 : Sum  Inputs=-+|
  Sum3 : Sum  Inputs=-+|
  Sum4 : Sum  Inputs=++|
  Sum5 : Sum  Inputs=|++
  Sum7 : Sum  Inputs=++|
  Sum9 : Sum  Inputs=++|
  C(nu_r)nu_r(4) : Outport
  wires:
  [v] -> Product4/2
  Product4/1 -> Gain13/1
  Product/1 -> Gain11/1
  [v] -> Product/2
  Gain11/1 -> Sum7/2
  [u] -> Product4/1
  Sum9/1 -> C(nu_r)nu_r(4)/1
  psi/1 -> Sin/1, Cos/1
  Sin/1 -> [sinpsi]
  Cos/1 -> [cospsi]
  u/1 -> [u]
  V_x/1 -> [V_x]
  V_y/1 -> [V_y]
  v/1 -> [v]
  Gain13/1 -> Sum9/1
  [V_y] -> Product1/1
  [V_x] -> Product5/2
  Product1/1 -> Sum/1
  Product5/1 -> Sum/2
  Sum/1 -> Product/1
  [sinpsi] -> Product1/2
  [cospsi] -> Product5/1
  Product2/1 -> Gain1/1
  [u] -> Product2/2
  [V_x] -> Product6/2
  Sum1/1 -> Product2/1
  [cospsi] -> Product3/2
  [V_y] -> Product3/1
  [sinpsi] -> Product6/1
  Product3/1 -> Sum1/1
  Product6/1 -> Sum1/2
  Gain1/1 -> Sum7/1
  [sinpsi] -> Product7/4
  [cospsi] -> Product7/3
  [V_x] -> Product7/1
  [V_x] -> Product7/2
  [sinpsi] -> Product9/4
  [V_y] -> Product9/1
  [cospsi] -> Product9/3
  [V_y] -> Product9/2
  Product7/1 -> Sum2/2
  Product9/1 -> Sum2/1
  [V_y] -> Product8/2
  [cospsi] -> Product8/3
  [V_x] -> Product8/1
  Product8/1 -> Sum3/1
  [cospsi] -> Product8/4
  [V_y] -> Product10/2
  [sinpsi] -> Product10/3
  [V_x] -> Product10/1
  [sinpsi] -> Product10/4
  Product10/1 -> Sum3/2
  Sum3/1 -> Sum4/2
  Sum2/1 -> Sum4/1
  Sum4/1 -> Gain2/1
  Sum7/1 -> Sum5/2
  Sum5/1 -> Sum9/2
  Gain2/1 -> Sum5/1

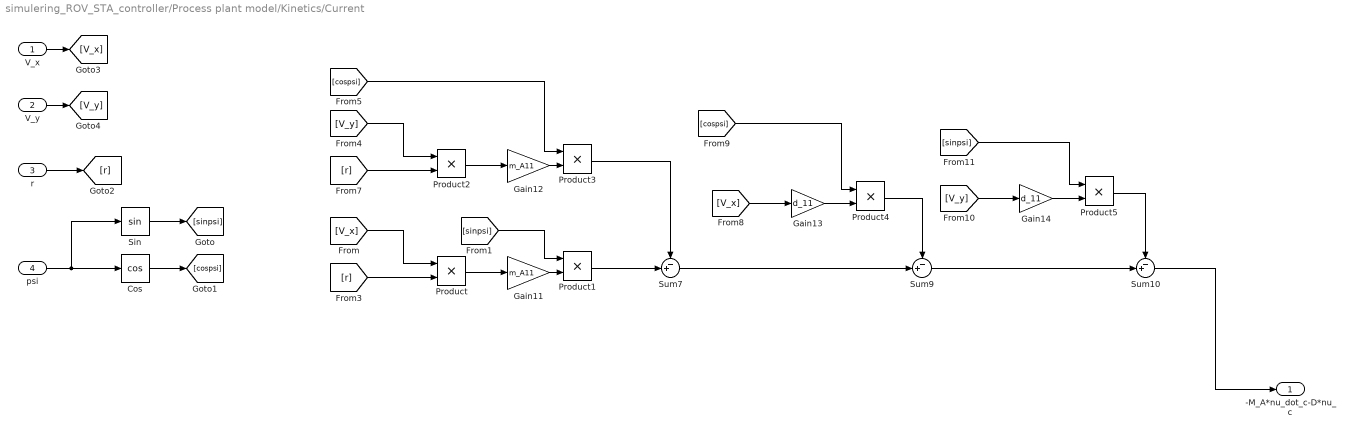
== system simulering_ROV_STA_controller/Process plant model/Kinetics/Current ==
  V_x : Inport
  V_y : Inport  Port=2
  r : Inport  Port=3
  psi : Inport  Port=4
  Cos : Trigonometry  Operator=cos
  Gain11 : Gain  Gain=m_A11
  Gain12 : Gain  Gain=m_A11
  Gain13 : Gain  Gain=d_11
  Gain14 : Gain  Gain=d_11
  Product{,1..5} (6 alike) : Product
  Sin : Trigonometry
  Sum10 : Sum  Inputs=-+|
  Sum7 : Sum  Inputs=-+|
  Sum9 : Sum  Inputs=-+|
  -M_A*nu_dot_c-D*nu_c : Outport
  wires:
  Gain11/1 -> Product1/2
  Product2/1 -> Gain12/1
  [cospsi] -> Product3/1
  [r] -> Product2/2
  Gain13/1 -> Product4/2
  Product4/1 -> Sum9/1
  [V_x] -> Product/1
  Product3/1 -> Sum7/1
  Gain12/1 -> Product3/2
  Product/1 -> Gain11/1
  [V_y] -> Product2/1
  [r] -> Product/2
  Product1/1 -> Sum7/2
  [sinpsi] -> Product1/1
  Gain14/1 -> Product5/2
  [sinpsi] -> Product5/1
  Sum7/1 -> Sum9/2
  [cospsi] -> Product4/1
  [V_y] -> Gain14/1
  [V_x] -> Gain13/1
  Product5/1 -> Sum10/1
  Sum9/1 -> Sum10/2
  Sum10/1 -> -M_A*nu_dot_c-D*nu_c/1
  psi/1 -> Sin/1, Cos/1
  Sin/1 -> [sinpsi]
  Cos/1 -> [cospsi]
  r/1 -> [r]
  V_x/1 -> [V_x]
  V_y/1 -> [V_y]

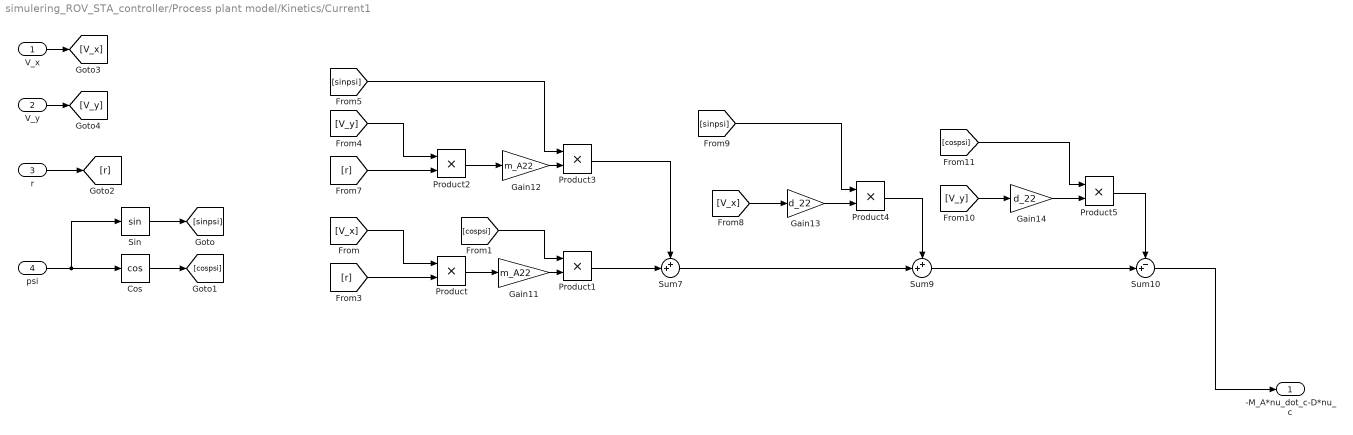
== system simulering_ROV_STA_controller/Process plant model/Kinetics/Current1 ==
  V_x : Inport
  V_y : Inport  Port=2
  r : Inport  Port=3
  psi : Inport  Port=4
  Cos : Trigonometry  Operator=cos
  Gain11 : Gain  Gain=m_A22
  Gain12 : Gain  Gain=m_A22
  Gain13 : Gain  Gain=d_22
  Gain14 : Gain  Gain=d_22
  Product{,1..5} (6 alike) : Product
  Sin : Trigonometry
  Sum10 : Sum  Inputs=-+|
  Sum7 : Sum  Inputs=++|
  Sum9 : Sum  Inputs=++|
  -M_A*nu_dot_c-D*nu_c : Outport
  wires:
  Gain11/1 -> Product1/2
  Product2/1 -> Gain12/1
  [sinpsi] -> Product3/1
  [r] -> Product2/2
  Gain13/1 -> Product4/2
  Product4/1 -> Sum9/1
  [V_x] -> Product/1
  Product3/1 -> Sum7/1
  Gain12/1 -> Product3/2
  Product/1 -> Gain11/1
  [V_y] -> Product2/1
  [r] -> Product/2
  Product1/1 -> Sum7/2
  [cospsi] -> Product1/1
  Gain14/1 -> Product5/2
  [cospsi] -> Product5/1
  Sum7/1 -> Sum9/2
  [sinpsi] -> Product4/1
  [V_y] -> Gain14/1
  [V_x] -> Gain13/1
  Product5/1 -> Sum10/1
  Sum9/1 -> Sum10/2
  Sum10/1 -> -M_A*nu_dot_c-D*nu_c/1
  psi/1 -> Sin/1, Cos/1
  Sin/1 -> [sinpsi]
  Cos/1 -> [cospsi]
  r/1 -> [r]
  V_x/1 -> [V_x]
  V_y/1 -> [V_y]

== system simulering_ROV_STA_controller/Process plant model/Kinetics/Nonlinear damping psi ==
  psi : Inport
  Abs : Abs
  Gain : Gain  Gain=d_n66
  Product : Product
  D_n(nu_r)nu_r(4) : Outport
  wires:
  Abs/1 -> Gain/1
  Product/1 -> D_n(nu_r)nu_r(4)/1
  Gain/1 -> Product/1
  psi/1 -> Abs/1, Product/2

== system simulering_ROV_STA_controller/Process plant model/Kinetics/Nonlinear damping u ==
  u : Inport
  V_x : Inport  Port=2
  V_y : Inport  Port=3
  psi : Inport  Port=4
  Abs : Abs
  Cos : Trigonometry  Operator=cos
  Gain : Gain  Gain=d_n11
  Product : Product
  Product4 : Product
  Product5 : Product
  Sin : Trigonometry
  Sum : Sum  Inputs=++|
  Sum1 : Sum  Inputs=-+|
  D_n(nu_r)nu_r(1) : Outport
  wires:
  Gain/1 -> Product/1
  Product/1 -> D_n(nu_r)nu_r(1)/1
  Abs/1 -> Gain/1
  psi/1 -> Sin/1, Cos/1
  Sin/1 -> [sinpsi]
  Cos/1 -> [cospsi]
  [V_y] -> Product5/2
  [sinpsi] -> Product5/1
  Product4/1 -> Sum/2
  [V_x] -> Product4/2
  [cospsi] -> Product4/1
  Product5/1 -> Sum/1
  V_x/1 -> [V_x]
  V_y/1 -> [V_y]
  u/1 -> Sum1/2
  Sum1/1 -> Product/2, Abs/1
  Sum/1 -> Sum1/1

== system simulering_ROV_STA_controller/Process plant model/Kinetics/Nonlinear damping v ==
  v : Inport
  V_x : Inport  Port=2
  V_y : Inport  Port=3
  psi : Inport  Port=4
  Abs : Abs
  Cos : Trigonometry  Operator=cos
  Gain : Gain  Gain=d_n22
  Product : Product
  Product4 : Product
  Product5 : Product
  Sin : Trigonometry
  Sum : Sum  Inputs=+-|
  Sum1 : Sum  Inputs=-+|
  D_n(nu_r)nu_r(2) : Outport
  wires:
  Gain/1 -> Product/1
  Product/1 -> D_n(nu_r)nu_r(2)/1
  Abs/1 -> Gain/1
  psi/1 -> Sin/1, Cos/1
  Sin/1 -> [sinpsi]
  Cos/1 -> [cospsi]
  [V_y] -> Product5/2
  Product4/1 -> Sum/2
  [V_x] -> Product4/2
  Product5/1 -> Sum/1
  V_x/1 -> [V_x]
  V_y/1 -> [V_y]
  v/1 -> Sum1/2
  Sum1/1 -> Product/2, Abs/1
  Sum/1 -> Sum1/1
  [sinpsi] -> Product4/1
  [cospsi] -> Product5/1

== system simulering_ROV_STA_controller/Process plant model/Kinetics/Nonlinear damping w ==
  w : Inport
  Abs : Abs
  Gain : Gain  Gain=d_n33
  Product : Product
  D_n(nu_r)nu_r(3) : Outport
  wires:
  Abs/1 -> Gain/1
  Product/1 -> D_n(nu_r)nu_r(3)/1
  Gain/1 -> Product/1
  w/1 -> Abs/1, Product/2

== matlab function simulering_ROV_STA_controller/Control law/Yaw controller/SSA ==
  data: u input; y output
function y = fcn(u)
%#codegen

y = ssa(u);

== matlab function simulering_ROV_STA_controller/MATLAB Function1 ==
  data: eta input size=4; V_mat input; V_actually output
function V_actually = fcn(eta, V_mat)
%#codegen
    x = eta(1);
    y = eta(2);
    
    V_actually = interp2(-2*50:2*50, -2*50:5*50, V_mat, x, y);

== matlab function simulering_ROV_STA_controller/MATLAB Function ==
  data: eta input size=4; V_mat input; Vx_actually output
function Vx_actually = fcn(eta, V_mat)
%#codegen
    x = eta(1);
    y = eta(2);
    
    Vx_actually = interp2(-2*50:2*50, -2*50:5*50, V_mat, x, y);
